simulink model "mc_mixer_old"  (R2021a)
settings: Solver=VariableStepAuto  StartTime=0.0  StopTime=10.0  RelTol=1e-3
undefined symbols (not defined in the file): DiscIntNeverNeededParam, MC_AIRMODE, THR_MDL_FAC
settings Model: DataDictionary=px4_dict.sldd  Creator=DELL  LastModifiedBy=DELL

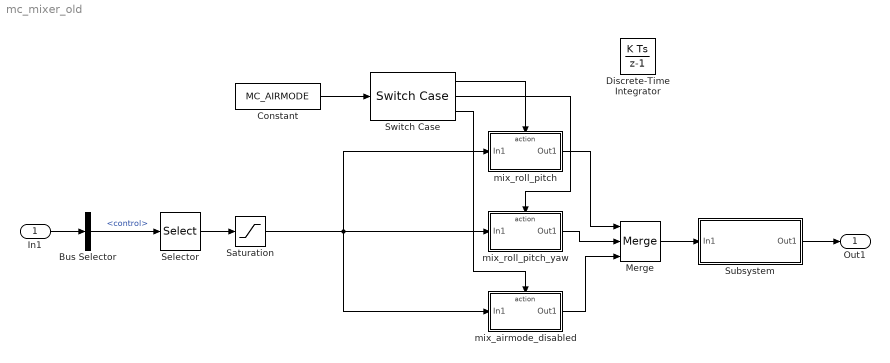
== system mc_mixer_old ==
  In1 : Inport  OutDataTypeStr=Bus: px4_actuator_controls
  Bus Selector : BusSelector  OutputSignals=control
  Constant : Constant  Value=MC_AIRMODE
  Discrete-Time Integrator : DiscreteIntegrator  ExternalReset=sampled level  InitialConditionSource=external  SampleTime=-1  ICPrevOutput=DiscIntNeverNeededParam  ICPrevScaledInput=DiscIntNeverNeededParam
  Merge : Merge  Inputs=3
  Saturation : Saturate
  Selector : Selector  InputPortWidth=3  IndexOptions=Index vector (dialog)  Indices=[1 3]  OutputSizes=1
  Subsystem : Subsystem
  Switch Case : SwitchCase  CaseConditions={1,2}
  mix_airmode_disabled : Subsystem  TreatAsAtomicUnit=on
  mix_roll_pitch : Subsystem  TreatAsAtomicUnit=on
  mix_roll_pitch_yaw : Subsystem  TreatAsAtomicUnit=on
  Out1 : Outport  OutDataTypeStr=Bus: px4_actuator_outputs
  wires:
  In1/1 -> Bus Selector/1
  Bus Selector/1 -> Selector/1  "<control>"
  Selector/1 -> Saturation/1
  Constant/1 -> Switch Case/1
  Switch Case/1 -> mix_roll_pitch/Action
  Switch Case/3 -> mix_airmode_disabled/Action
  Switch Case/2 -> mix_roll_pitch_yaw/Action
  mix_roll_pitch_yaw/1(Out1) -> Merge/2
  mix_airmode_disabled/1(Out1) -> Merge/3
  mix_roll_pitch/1(Out1) -> Merge/1
  Saturation/1 -> mix_roll_pitch/1(In1), mix_airmode_disabled/1(In1), mix_roll_pitch_yaw/1(In1)
  Merge/1 -> Subsystem/1(In1)
  Subsystem/1(Out1) -> Out1/1
  ? -> Discrete-Time Integrator/2
  ? -> Discrete-Time Integrator/3

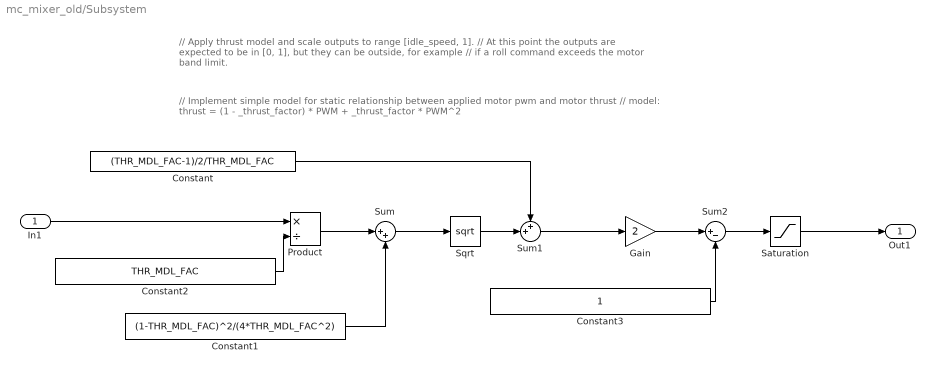
== system mc_mixer_old/Subsystem ==
  note: // Implement simple model for static relationship between applied motor pwm and motor thrust
      | // model: thrust = (1 - _thrust_factor) * PWM + _thrust_factor * PWM^2
  note: // Apply thrust model and scale outputs to range [idle_speed, 1].
      | // At this point the outputs are expected to be in [0, 1], but they can be outside, for example
      | // if a roll command exceeds the motor band limit.
  In1 : Inport
  Constant : Constant  Value=(THR_MDL_FAC-1)/2/THR_MDL_FAC
  Constant1 : Constant  Value=(1-THR_MDL_FAC)^2/(4*THR_MDL_FAC^2)
  Constant2 : Constant  Value=THR_MDL_FAC
  Constant3 : Constant
  Gain : Gain  Gain=2
  Product : Product  Inputs=*/
  Saturation : Saturate  UpperLimit=1  LowerLimit=-1
  Sqrt : Sqrt  SaturateOnIntegerOverflow=on
  Sum : Sum  Inputs=|++
  Sum1 : Sum  Inputs=++|
  Sum2 : Sum  Inputs=|+-
  Out1 : Outport
  wires:
  In1/1 -> Product/1
  Constant1/1 -> Sum/2
  Product/1 -> Sum/1
  Constant2/1 -> Product/2
  Sum/1 -> Sqrt/1
  Constant/1 -> Sum1/1
  Sqrt/1 -> Sum1/2
  Sum1/1 -> Gain/1
  Sum2/1 -> Saturation/1
  Gain/1 -> Sum2/1
  Constant3/1 -> Sum2/2
  Saturation/1 -> Out1/1

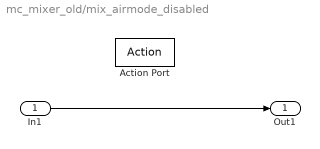
== system mc_mixer_old/mix_airmode_disabled ==
  In1 : Inport
  Action Port : ActionPort  ActionPortLabel=default:
  Out1 : Outport
  wires:
  In1/1 -> Out1/1

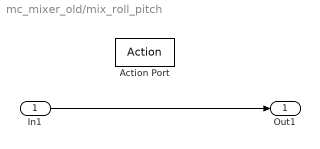
== system mc_mixer_old/mix_roll_pitch ==
  In1 : Inport
  Action Port : ActionPort  ActionPortLabel=case [ 1 ]:
  Out1 : Outport
  wires:
  In1/1 -> Out1/1

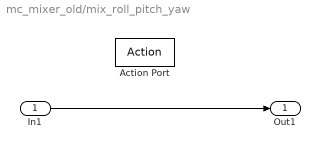
== system mc_mixer_old/mix_roll_pitch_yaw ==
  In1 : Inport
  Action Port : ActionPort  ActionPortLabel=case [ 2 ]:
  Out1 : Outport
  wires:
  In1/1 -> Out1/1
